simulink model "wnch_Notch_01"  (R2019b)
settings: Solver=FixedStepAuto  StartTime=0.0  StopTime=0.5  FixedStep=50e-6  MaxStep=1e-3  RelTol=1e-3
settings Model: Creator=wnch  LastModifiedBy=wnch

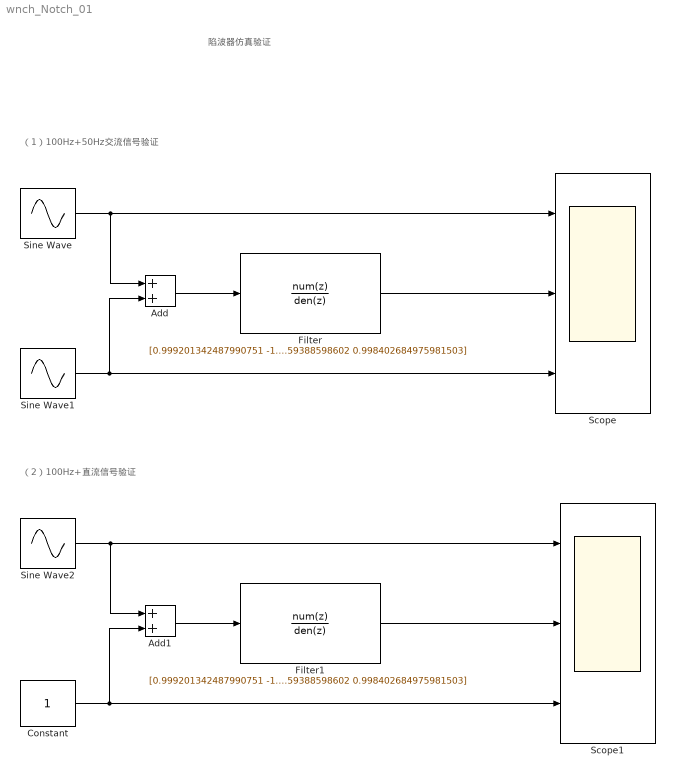
== system wnch_Notch_01 ==
  note: （1）100Hz+50Hz交流信号验证
  note: 陷波器仿真验证
  note: （2）100Hz+直流信号验证
  Add : Sum
  Add1 : Sum
  Constant : Constant
  Filter : DiscreteFilter  Tag=BlockMethodSubSystem  Numerator=[0.999201342487990751 -1.99741659388598602 0.999201342487990751]  Denominator=[1 -1.99741659388598602 0.998402684975981503]  InputProcessing=Columns as channels (frame based)  a0EqualsOne=on
  Filter1 : DiscreteFilter  Tag=BlockMethodSubSystem  Numerator=[0.999201342487990751 -1.99741659388598602 0.999201342487990751]  Denominator=[1 -1.99741659388598602 0.998402684975981503]  InputProcessing=Columns as channels (frame based)  a0EqualsOne=on
  Scope : Scope  NumInputPorts=3
  Scope1 : Scope  NumInputPorts=3
  Sine Wave : Sin  Frequency=100*2*pi  SampleTime=0
  Sine Wave1 : Sin  Frequency=50*2*pi  SampleTime=0
  Sine Wave2 : Sin  Frequency=100*2*pi  SampleTime=0
  wires:
  Sine Wave/1 -> Add/1, Scope/1
  Sine Wave1/1 -> Scope/3, Add/2
  Add/1 -> Filter/1
  Filter/1 -> Scope/2
  Sine Wave2/1 -> Scope1/1, Add1/1
  Add1/1 -> Filter1/1
  Constant/1 -> Scope1/3, Add1/2
  Filter1/1 -> Scope1/2
